simulink model "BDK_thich_nghi_luat_dk_ti_le"  (R2023a)
settings: Solver=VariableStepAuto  StartTime=0.0  StopTime=100  RelTol=1e-3
settings Model: Creator=VINH  LastModifiedBy=VINH

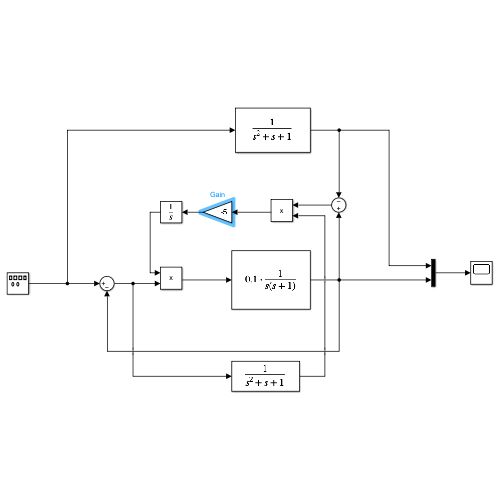
[thumbnail: Simulink's stored preview of the top-level diagram]
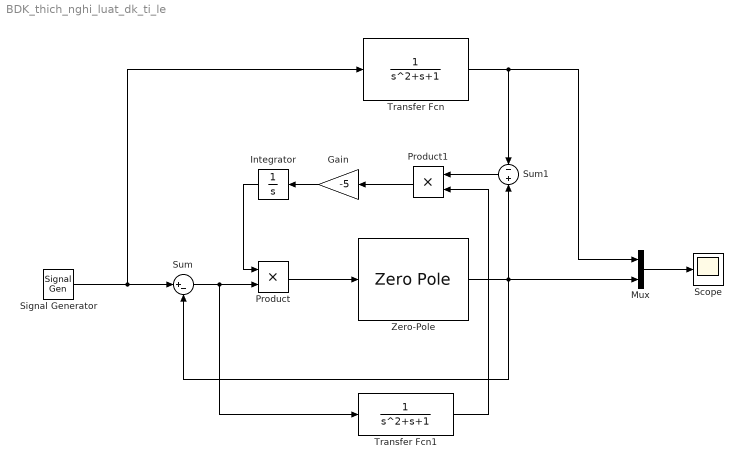
== system BDK_thich_nghi_luat_dk_ti_le ==
  Gain : Gain  Gain=-5
  Integrator : Integrator
  Mux : Mux  Inputs=2
  Product : Product
  Product1 : Product
  Scope : Scope
  Signal Generator : SignalGenerator  WaveForm=square  Amplitude=0.5  Frequency=0.1
  Sum : Sum  Inputs=|+-
  Sum1 : Sum  Inputs=-|+
  Transfer Fcn : TransferFcn  Denominator=[1 1 1]
  Transfer Fcn1 : TransferFcn  Denominator=[1 1 1]
  Zero-Pole : ZeroPole  Zeros=[]  Poles=[0 -1]  Gain=0.1
  wires:
  Product/1 -> Zero-Pole/1
  Sum/1 -> Product/2, Transfer Fcn1/1
  Signal Generator/1 -> Sum/1, Transfer Fcn/1
  Zero-Pole/1 -> Mux/2, Sum1/2, Sum/2
  Transfer Fcn/1 -> Mux/1, Sum1/1
  Transfer Fcn1/1 -> Product1/2
  Sum1/1 -> Product1/1
  Product1/1 -> Gain/1
  Gain/1 -> Integrator/1
  Integrator/1 -> Product/1
  Mux/1 -> Scope/1
